simulink model "Lab6_Fuzzy"  (R2020a)
settings: Solver=VariableStepAuto  StartTime=0.0  StopTime=1000  RelTol=1e-3
libraries: fuzblock x1
settings Model: Creator=mitch  LastModifiedBy=mitch

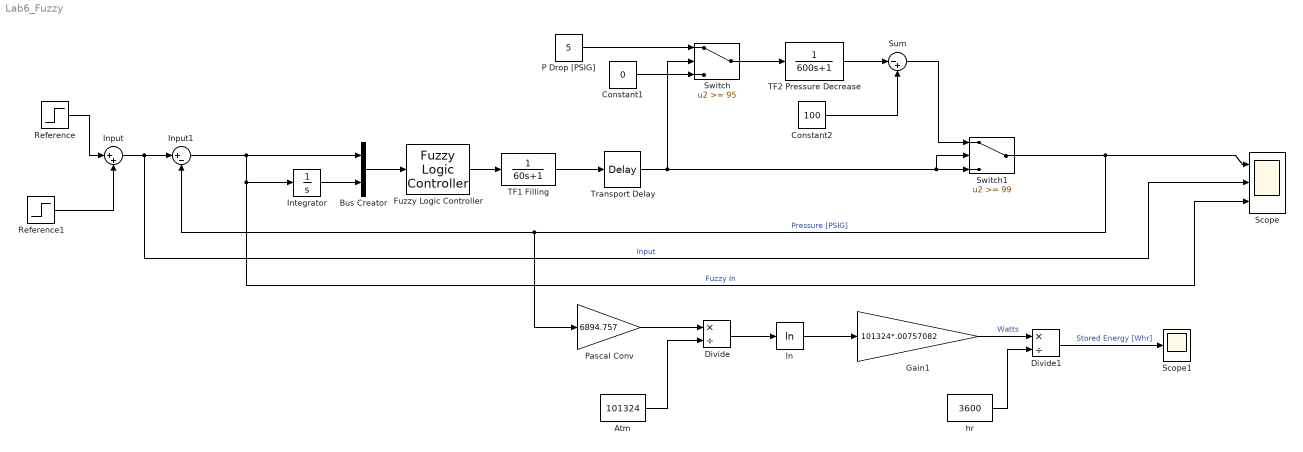
== system Lab6_Fuzzy ==
  Atm : Constant  Value=101324
  Bus Creator : BusCreator  Inputs=2
  Constant1 : Constant  Value=0
  Constant2 : Constant  Value=100
  Divide : Product  Inputs=*/
  Divide1 : Product  Inputs=*/
  Fuzzy Logic Controller : fuzblock/Fuzzy Logic  Controller  FIS='lab6.fis'  OutputSampleNumber=101  DataType=double  FuzzifiedInputs=off  RuleFiringStrengths=off  RuleOutputs=off  AggregatedOutputs=off  SimulateUsing=Interpreted execution  OutOfRangeInputValueMessage=warning  NoRuleFiredMessage=warning  EmptyOutputFuzzySetMessage=warning
  Gain1 : Gain  Gain=101324*.00757082
  Input : Sum  Inputs=|++
  Input1 : Sum  Inputs=|+-
  Integrator : Integrator
  P Drop [PSIG] : Constant  Value=5
  Pascal Conv : Gain  Gain=6894.757
  Reference : Step  Time=10  After=60  SampleTime=0
  Reference1 : Step  Time=500  After=40  SampleTime=0
  Scope : Scope  NumInputPorts=3
  Scope1 : Scope
  Sum : Sum  Inputs=|-+
  Switch : Switch  Threshold=95
  Switch1 : Switch  Threshold=99
  TF1 Filling : TransferFcn  Denominator=[60 1]
  TF2 Pressure Decrease : TransferFcn  Denominator=[600 1]
  Transport Delay : TransportDelay
  hr : Constant  Value=3600
  ln : Math  Operator=log  SaturateOnIntegerOverflow=on
  wires:
  Constant2/1 -> Sum/2
  TF2 Pressure Decrease/1 -> Sum/1
  Pascal Conv/1 -> Divide/1
  Atm/1 -> Divide/2
  Divide/1 -> ln/1
  ln/1 -> Gain1/1
  Gain1/1 -> Divide1/1  "Watts"
  hr/1 -> Divide1/2
  TF1 Filling/1 -> Transport Delay/1
  P Drop [PSIG]/1 -> Switch/1
  Transport Delay/1 -> Switch/2, Switch1/2, Switch1/3
  Constant1/1 -> Switch/3
  Switch/1 -> TF2 Pressure Decrease/1
  Sum/1 -> Switch1/1
  Switch1/1 -> Input1/2, Pascal Conv/1, Scope/1  "Pressure [PSIG]"
  Reference/1 -> Input/1
  Fuzzy Logic Controller/1 -> TF1 Filling/1
  Divide1/1 -> Scope1/1  "Stored Energy [Whr]"
  Reference1/1 -> Input/2
  Input/1 -> Scope/2, Input1/1  "Input"
  Bus Creator/1 -> Fuzzy Logic Controller/1
  Integrator/1 -> Bus Creator/2
  Input1/1 -> Scope/3, Integrator/1, Bus Creator/1  "Fuzzy In"
